simulink model "hexapod"  (R2015a)
settings: Solver=ode23tb  StartTime=0.0  StopTime=10  FixedStep=0.001  MaxStep=0.01  RelTol=1e-4  AbsTol=1e-5
values from neighbouring files (symbols this model uses):
  bL = 18.5    [runFirst.m]    (also in runFirst2.m = 20.5)
  bWb = 12.5    [runFirst.m]    (also in runFirst2.m = 14.5)
  bWs = 10.5    [runFirst.m]    (also in runFirst2.m = 12.5)
  C = CM + CL/n^2    (= 0.0001377500155)    [runFirst.m]
  d1 = 0    [runFirst.m]    (also in runFirst2.m)
  d2 = -4.61    [runFirst.m]    (also in runFirst2.m = 0)
  J = JM + JL/n^2    (= 0.008455500031)    [runFirst.m]
  Ka = 12    [runFirst.m]
  Kb = 0.00867    [runFirst.m]
  Ke = 1    [runFirst.m]
  Km = 4.375    [runFirst.m]
  L = 0.0006    [runFirst.m]
  L1 = 3.64    [runFirst.m]    (also in runFirst2.m = 3.4)
  l1x = 15.78    [runFirst.m]
  l1y = 11.78    [runFirst.m]
  l1z = -14.9    [runFirst.m]
  L2 = 5.72    [runFirst.m]    (also in runFirst2.m = 8.7)
  l2x = 0    [runFirst.m]
  l2y = 15.48    [runFirst.m]
  l2z = -14.9    [runFirst.m]
  L3 = 12.46    [runFirst.m]    (also in runFirst2.m = 12.73)
  l3x = -15.78    [runFirst.m]
  l3y = 11.78    [runFirst.m]
  l3z = -14.9    [runFirst.m]
  l4x = 15.78    [runFirst.m]
  l4y = -11.78    [runFirst.m]
  l4z = -14.9    [runFirst.m]
  l5x = 0    [runFirst.m]
  l5y = -15.48    [runFirst.m]
  l5z = -14.9    [runFirst.m]
  l6x = -15.78    [runFirst.m]
  l6y = -11.78    [runFirst.m]
  l6z = -14.9    [runFirst.m]
  n = 254    [runFirst.m]
  R = 1.4    [runFirst.m]
  stX = 4    [runFirst.m]
  stZ = 2    [runFirst.m]
  Ts = 2    [runFirst.m]
undefined symbols (not defined in the file or in its folder): X, Y, Z
undefined symbols (not defined in the file): bH, bM, m1, m2, m3
libraries: sm_lib x108, nesl_utility x52, simulink x12, Contact_Forces_Lib x7, roblocks x2
(part 1 of 5)
settings Model: Creator=340DANILOV  LastModifiedBy=340DANILOV
settings SolverCC: ZeroCrossAlgorithm=Adaptive
settings DataIOCC: LimitDataPoints=off  ReturnWorkspaceOutputs=on
settings DebuggingCC: IgnoredZcDiagnostic=none  SolverPrmCheckMsg=warning  UnconnectedInputMsg=none  UnconnectedOutputMsg=none
settings DiagnosticsConfigSet: SimMechanicsRigidlyBoundBlock=none

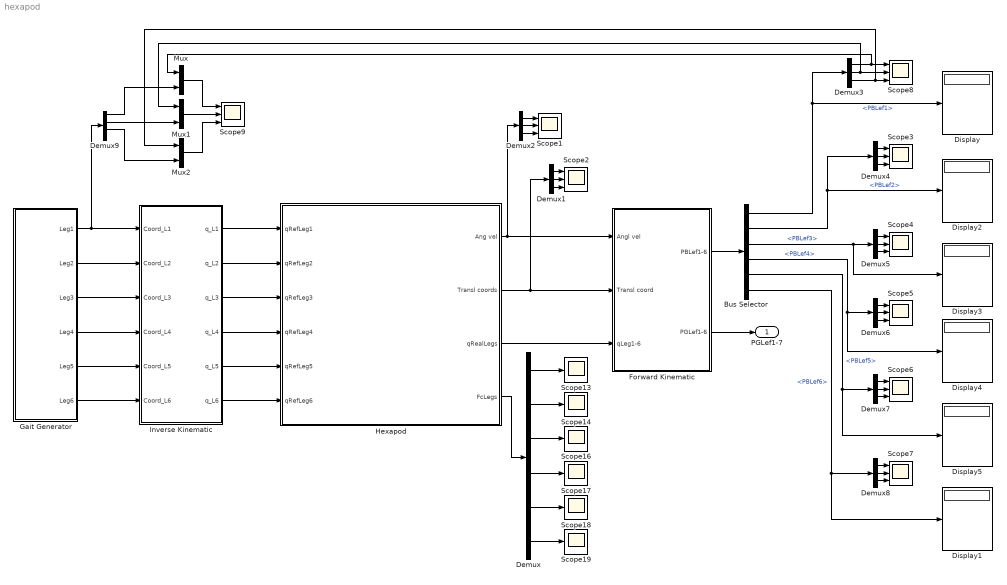
== system hexapod ==
  Bus Selector : BusSelector  OutputSignals=PBLef1,PBLef2,PBLef3,PBLef4,PBLef5,PBLef6
  Demux : Demux  Outputs=6
  Demux{1..8} (8 alike) : Demux  Outputs=3
  Demux9 : Demux
  Display{,1..5} (6 alike) : Display
  Forward Kinematic : Subsystem
  Gait Generator : Subsystem
  Hexapod : Subsystem  mask(Hexapod model){bLength=bL, bSmWidth=bWs, bBigWidth=bWb, bHeight=bH, bMass=bM, L1Length=L1, L2Length=L2, L3Length=L3, L1Mass=m1, L2Mass=m2, L3Mass=m3, dirAngle=45, GsurfX=10, GsurfY=1}
      mask prompts: bLength "Length [cm]"; bSmWidth "Small Width  [cm]"; bBigWidth "Big Width  [cm]"; bHeight "Height  [cm]"; bMass "Mass [kg]"; L1Length "Link 1"; L2Length "Link 2"; L3Length "Link3"; L1Mass "Link 1"; L2Mass "Link 2"; L3Mass "Link 3"; dirAngle "Angle of legs direction relative to body [grad]"; GsurfX "X"; GsurfY "Y"
      mask help:
      | This model describes hexapod robot with six insect legs. This model contain mechanics and servos.
      | You can change mass and size charasteristics of body and legs.
      | As a location is used a flat surface.
      |
      | Inputs:
      |  - qRefLeg<1...6> - reference angles for each leg.
      |             It is must be 1x3 massive with angles for each joint of leg.
      |
      | Outputs:
      |  - Ang vel - Angular velocities of CoM. Imitation of data from gyroscope.
      |  - Transl accel - CoM translation acceleration. Imitation of data from accelerometer.
      |  - FcLegs - Contact forces of end effectors each leg. It is 1x6 massive. Each element contains value for contact force each leg. Imitation of force sensors.
      |  - qRealLegs - Real angles of each link of hexapod legs. It is 3x6 massive. Imitation of data from servo encoder.
      mask DialogControl Control2 Prompt: You can customize parameters of the hexapod body here.
      mask DialogControl Container8 Prompt: Length of links [cm]
      mask DialogControl Container14 Prompt: Mass of links [kg]
      mask DialogControl Control6 Prompt: Enter parameters of surface geometry [m].
      mask Display:
      | image(imread('hexapod.png'))
      | 
      | 
      | port_label('output',1,'Ang vel')
      | port_label('output',2,'Transl accel')
      | port_label('output',3,'qRealLegs')
      | port_label('output',4,'FcLegs')
      | 
      | port_label('input',1,'qRefLeg1')
      | port_label('input',2,'qRefLeg2')
      | port_label('input',3,'qRefLeg3')
      | port_label('input',4,'qRefLeg4')
      | port_label('input',5,'qRefLeg5')
      | port_label('input',6,'qRefLeg6')
  Inverse Kinematic : Subsystem
  Mux : Mux  Inputs=2
  Mux1 : Mux  Inputs=2
  Mux2 : Mux  Inputs=2
  Scope{1..9} (9 alike) : Scope  NumInputPorts=3
      Scope1 settings: YMin=-15~-5~-5  YMax=20~5~5  SaveName=ScopeData22
      Scope2 settings: YMin=-15~-5~-5  YMax=20~5~5  SaveName=ScopeData25
      Scope3 settings: YMin=-15~-5~-5  YMax=20~5~5  SaveName=ScopeData32
      Scope4 settings: YMin=-15~-5~-5  YMax=20~5~5  SaveName=ScopeData33
      Scope5 settings: YMin=-15~-5~-5  YMax=20~5~5  SaveName=ScopeData34
      Scope6 settings: YMin=-15~-5~-5  YMax=20~5~5  SaveName=ScopeData35
      Scope7 settings: YMin=-15~-5~-5  YMax=20~5~5  SaveName=ScopeData36
      Scope8 settings: YMin=-15~-5~-5  YMax=20~5~5  SaveName=ScopeData44
      Scope9 settings: YMin=-15~10.5~-5  YMax=20~13~5  SaveName=ScopeData37
  Scope{13..14,16..19} (6 alike) : Scope
      Scope13 settings: SaveName=ScopeData23
      Scope14 settings: SaveName=ScopeData24
      Scope16 settings: SaveName=ScopeData26
      Scope17 settings: SaveName=ScopeData27
      Scope18 settings: SaveName=ScopeData28
      Scope19 settings: SaveName=ScopeData29
  PGLef1-7 : Outport
  wires:
  Hexapod/4(FcLegs) -> Demux/1
  Hexapod/1(Ang vel) -> Demux2/1, Forward Kinematic/1(Angl vel)
  Hexapod/2(Transl coords) -> Demux1/1, Forward Kinematic/2(Transl coord)
  Hexapod/3(qRealLegs) -> Forward Kinematic/3(qLeg1-6)
  Forward Kinematic/1(PBLef1-6) -> Bus Selector/1
  Forward Kinematic/2(PGLef1-6) -> PGLef1-7/1
  Bus Selector/1 -> Demux3/1, Display/1  "<PBLef1>"
  Bus Selector/6 -> Demux8/1, Display1/1  "<PBLef6>"
  Bus Selector/2 -> Demux4/1, Display2/1  "<PBLef2>"
  Bus Selector/3 -> Demux5/1, Display3/1  "<PBLef3>"
  Bus Selector/4 -> Demux6/1, Display4/1  "<PBLef4>"
  Bus Selector/5 -> Demux7/1, Display5/1  "<PBLef5>"
  Gait Generator/2(Leg2) -> Inverse Kinematic/2(Coord_L2)
  Gait Generator/1(Leg1) -> Demux9/1, Inverse Kinematic/1(Coord_L1)
  Gait Generator/3(Leg3) -> Inverse Kinematic/3(Coord_L3)
  Gait Generator/4(Leg4) -> Inverse Kinematic/4(Coord_L4)
  Gait Generator/5(Leg5) -> Inverse Kinematic/5(Coord_L5)
  Gait Generator/6(Leg6) -> Inverse Kinematic/6(Coord_L6)
  Inverse Kinematic/2(q_L2) -> Hexapod/2(qRefLeg2)
  Inverse Kinematic/1(q_L1) -> Hexapod/1(qRefLeg1)
  Inverse Kinematic/3(q_L3) -> Hexapod/3(qRefLeg3)
  Inverse Kinematic/4(q_L4) -> Hexapod/4(qRefLeg4)
  Inverse Kinematic/5(q_L5) -> Hexapod/5(qRefLeg5)
  Inverse Kinematic/6(q_L6) -> Hexapod/6(qRefLeg6)
  Demux/1 -> Scope13/1
  Demux/2 -> Scope14/1
  Demux/3 -> Scope16/1
  Demux/4 -> Scope17/1
  Demux/5 -> Scope18/1
  Demux/6 -> Scope19/1
  Demux2/3 -> Scope1/3
  Demux2/2 -> Scope1/2
  Demux2/1 -> Scope1/1
  Demux1/3 -> Scope2/3
  Demux1/2 -> Scope2/2
  Demux1/1 -> Scope2/1
  Demux3/1 -> Scope8/1, Mux/1
  Demux4/3 -> Scope3/3
  Demux4/2 -> Scope3/2
  Demux4/1 -> Scope3/1
  Demux5/3 -> Scope4/3
  Demux5/2 -> Scope4/2
  Demux5/1 -> Scope4/1
  Demux6/3 -> Scope5/3
  Demux6/2 -> Scope5/2
  Demux6/1 -> Scope5/1
  Demux7/3 -> Scope6/3
  Demux7/2 -> Scope6/2
  Demux7/1 -> Scope6/1
  Demux8/3 -> Scope7/3
  Demux8/2 -> Scope7/2
  Demux8/1 -> Scope7/1
  Demux9/1 -> Mux/2
  Demux9/2 -> Mux1/2
  Demux9/3 -> Mux2/2
  Demux3/2 -> Scope8/2, Mux1/1
  Demux3/3 -> Scope8/3, Mux2/1
  Mux1/1 -> Scope9/2
  Mux/1 -> Scope9/1
  Mux2/1 -> Scope9/3

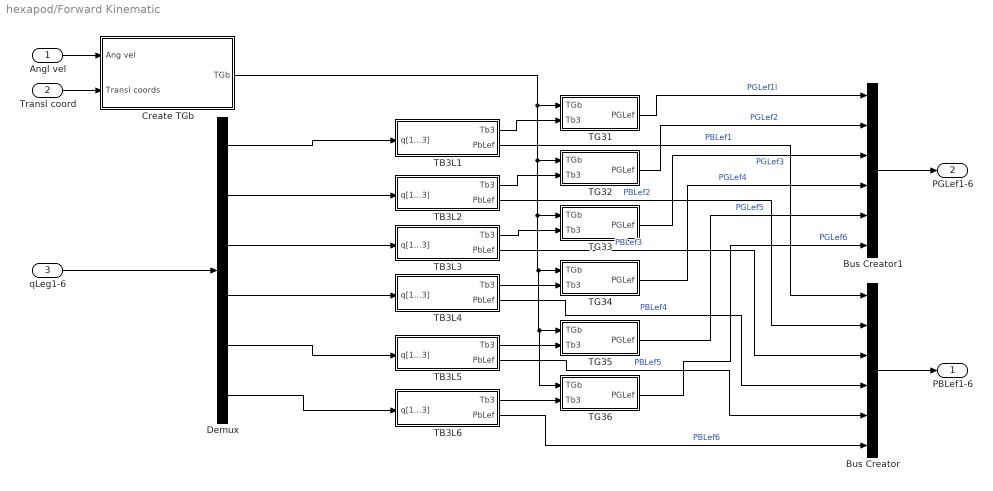
== system hexapod/Forward Kinematic ==
  Angl vel : Inport
  Transl coord : Inport  Port=2
  qLeg1-6 : Inport  Port=3
  Bus Creator : BusCreator  Inputs=6
  Bus Creator1 : BusCreator  Inputs=6
  Create TGb : Subsystem
  Demux : Demux  Outputs=6
  TB3L1 : Subsystem
  TB3L2 : Subsystem
  TB3L3 : Subsystem
  TB3L4 : Subsystem
  TB3L5 : Subsystem
  TB3L6 : Subsystem
  TG31 : Subsystem
  TG32 : Subsystem
  TG33 : Subsystem
  TG34 : Subsystem
  TG35 : Subsystem
  TG36 : Subsystem
  PBLef1-6 : Outport
  PGLef1-6 : Outport  Port=2
  wires:
  Bus Creator/1 -> PBLef1-6/1
  TB3L6/1(Tb3) -> TG36/2(Tb3)
  TB3L5/2(PbLef) -> Bus Creator/5  "PBLef5"
  TB3L4/2(PbLef) -> Bus Creator/4  "PBLef4"
  TG35/1(PGLef) -> Bus Creator1/5  "PGLef5"
  TB3L6/2(PbLef) -> Bus Creator/6  "PBLef6"
  Demux/1 -> TB3L1/1(q[1...3])
  TB3L1/2(PbLef) -> Bus Creator/1  "PBLef1"
  Demux/6 -> TB3L6/1(q[1...3])
  TB3L1/1(Tb3) -> TG31/2(Tb3)
  Create TGb/1(TGb) -> TG36/1(TGb), TG35/1(TGb), TG34/1(TGb), TG33/1(TGb), TG32/1(TGb), TG31/1(TGb)
  Demux/4 -> TB3L4/1(q[1...3])
  Demux/3 -> TB3L3/1(q[1...3])
  TG31/1(PGLef) -> Bus Creator1/1  "PGLef1l"
  Demux/5 -> TB3L5/1(q[1...3])
  TB3L2/2(PbLef) -> Bus Creator/2  "PBLef2"
  TB3L2/1(Tb3) -> TG32/2(Tb3)
  TG32/1(PGLef) -> Bus Creator1/2  "PGLef2"
  TB3L4/1(Tb3) -> TG34/2(Tb3)
  TB3L3/1(Tb3) -> TG33/2(Tb3)
  TG33/1(PGLef) -> Bus Creator1/3  "PGLef3"
  Bus Creator1/1 -> PGLef1-6/1
  Angl vel/1 -> Create TGb/1(Ang vel)
  Transl coord/1 -> Create TGb/2(Transl coords)
  TB3L3/2(PbLef) -> Bus Creator/3  "PBLef3"
  qLeg1-6/1 -> Demux/1
  TB3L5/1(Tb3) -> TG35/2(Tb3)
  TG36/1(PGLef) -> Bus Creator1/6  "PGLef6"
  TG34/1(PGLef) -> Bus Creator1/4  "PGLef4"
  Demux/2 -> TB3L2/1(q[1...3])

== system hexapod/Gait Generator ==
  Leg1_xyz : Subsystem
  Leg2_xyz : Subsystem
  Leg3_xyz : Subsystem
  Leg4_xyz : Subsystem
  Leg5_xyz : Subsystem
  Leg6_xyz : Subsystem
  Leg1 : Outport
  Leg2 : Outport  Port=2
  Leg3 : Outport  Port=3
  Leg4 : Outport  Port=4
  Leg5 : Outport  Port=5
  Leg6 : Outport  Port=6
  wires:
  Leg6_xyz/1(Out1) -> Leg6/1
  Leg1_xyz/1(Out1) -> Leg1/1
  Leg5_xyz/1(Out1) -> Leg5/1
  Leg3_xyz/1(Out1) -> Leg3/1
  Leg2_xyz/1(Out1) -> Leg2/1
  Leg4_xyz/1(Out1) -> Leg4/1

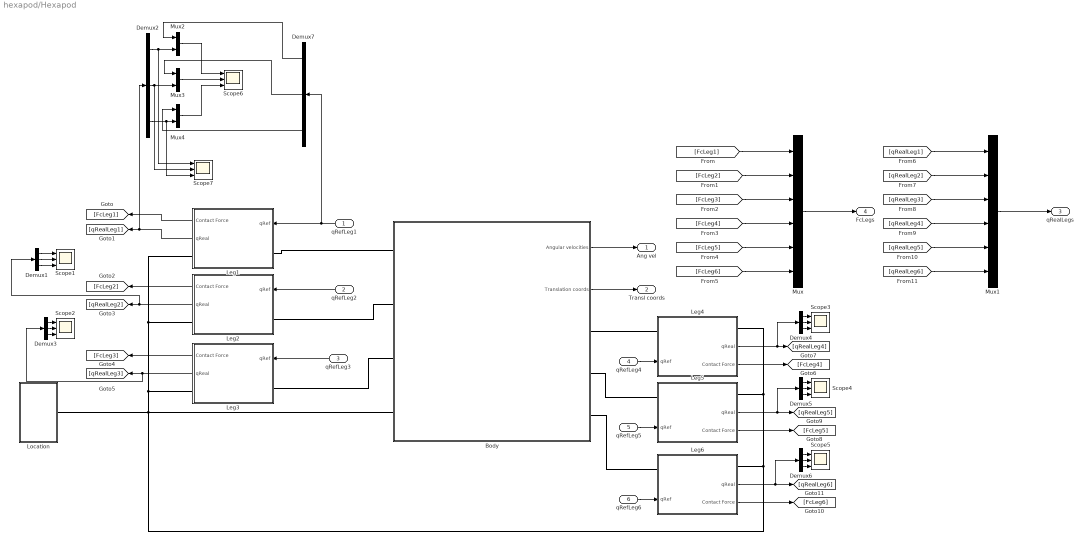
== system hexapod/Hexapod ==
  qRefLeg1 : Inport
  qRefLeg2 : Inport  Port=2
  qRefLeg3 : Inport  Port=3
  qRefLeg4 : Inport  Port=4
  qRefLeg5 : Inport  Port=5
  qRefLeg6 : Inport  Port=6
  Body : Subsystem  mask(Hexapod Body){L=bLength, w1=bSmWidth, w2=bBigWidth, H=bHeight, m=bMass, Z1Angle=dirAngle, Z2Angle=0, Z3Angle=-dirAngle, Z4Angle=-dirAngle, Z5Angle=0, Z6Angle=dirAngle}
      mask prompts: L "Length (cm)"; w1 "Small weigth (cm)"; w2 "Big weigth (cm)"; H "Heigth (cm)"; m "Mass (kg)"; Z1Angle "Leg1 Rotation"; Z2Angle "Leg2 Rotation"; Z3Angle "Leg3 Rotation"; Z4Angle "Leg4 Rotation"; Z5Angle "Leg5 Rotation"; Z6Angle "Leg6 Rotation"
      mask help: This block describes overall size, mass and reference frames of hexapod body.
      mask Display:
      | image(imread('body.png'))
      | text(5,10, 'Hexapod Body')
      | port_label('LConn',1,'Leg1')
      | port_label('LConn',2,'Leg2')
      | port_label('LConn',3,'Leg3')
      | port_label('LConn',4,'Global System')
      | port_label('RConn',1,'Leg4')
      | port_label('RConn',2,'Leg5')
      | port_label('RConn',3,'Leg6')
      | port_label('output',1,'Ang vel')
      | port_label('output',2,'Transl accel')
  Demux{1..7} (7 alike) : Demux  Outputs=3
  Leg1 : Subsystem  mask(Insect leg){L1=L1Length, L2=L2Length, L3=L3Length, m1=L1Mass, m2=L2Mass, m3=L3Mass}
      mask prompts: L1 "Length 1 (cm)"; L2 "Lengh 2 (cm)"; L3 "Length 3 (cm)"; m1 "Mass 1 (kg)"; m2 "Mass 2 (kg)"; m3 "Mass 3(kg)"
      mask help: This block describes link length and their mass of the hexapod insect leg.
      mask Display:
      | image(imread('insect_leg.png'))
      | text(5,10, 'Insect leg')
      | port_label('LConn',1,'T0')
      | port_label('RConn',1,'Base')
      | port_label('input',1,'qRef')
      | port_label('output',1,'Fc')
      | port_label('output',2,'qReal')
  Leg2 : Subsystem  mask(Insect leg){L1=L1Length, L2=L2Length, L3=L3Length, m1=L1Mass, m2=L2Mass, m3=L3Mass}
      mask prompts: L1 "Length 1 (cm)"; L2 "Lengh 2 (cm)"; L3 "Length 3 (cm)"; m1 "Mass 1 (kg)"; m2 "Mass 2 (kg)"; m3 "Mass 3(kg)"
      mask help: This block describes link length and their mass of the hexapod insect leg.
      mask Display:
      | image(imread('insect_leg.png'))
      | text(5,10, 'Insect leg')
      | port_label('LConn',1,'T0')
      | port_label('RConn',1,'Base')
      | port_label('input',1,'qRef')
      | port_label('output',1,'Fc')
      | port_label('output',2,'qReal')
  Leg3 : Subsystem  mask(Insect leg){L1=L1Length, L2=L2Length, L3=L3Length, m1=L1Mass, m2=L2Mass, m3=L3Mass}
      mask prompts: L1 "Length 1 (cm)"; L2 "Lengh 2 (cm)"; L3 "Length 3 (cm)"; m1 "Mass 1 (kg)"; m2 "Mass 2 (kg)"; m3 "Mass 3(kg)"
      mask help: This block describes link length and their mass of the hexapod insect leg.
      mask Display:
      | image(imread('insect_leg.png'))
      | text(5,10, 'Insect leg')
      | port_label('LConn',1,'T0')
      | port_label('RConn',1,'Base')
      | port_label('input',1,'qRef')
      | port_label('output',1,'Fc')
      | port_label('output',2,'qReal')
  Leg4 : Subsystem  mask(Insect leg){L1=L1Length, L2=L2Length, L3=L3Length, m1=L1Mass, m2=L2Mass, m3=L3Mass}
      mask prompts: L1 "Length 1 (cm)"; L2 "Lengh 2 (cm)"; L3 "Length 3 (cm)"; m1 "Mass 1 (kg)"; m2 "Mass 2 (kg)"; m3 "Mass 3(kg)"
      mask help: This block describes link length and their mass of the hexapod insect leg.
      mask Display:
      | image(imread('insect_leg.png'))
      | text(5,10, 'Insect leg')
      | port_label('LConn',1,'T0')
      | port_label('RConn',1,'Base')
      | port_label('input',1,'qRef')
      | port_label('output',1,'Fc')
      | port_label('output',2,'qReal')
  Leg5 : Subsystem  mask(Insect leg){L1=L1Length, L2=L2Length, L3=L3Length, m1=L1Mass, m2=L2Mass, m3=L3Mass}
      mask prompts: L1 "Length 1 (cm)"; L2 "Lengh 2 (cm)"; L3 "Length 3 (cm)"; m1 "Mass 1 (kg)"; m2 "Mass 2 (kg)"; m3 "Mass 3(kg)"
      mask help: This block describes link length and their mass of the hexapod insect leg.
      mask Display:
      | image(imread('insect_leg.png'))
      | text(5,10, 'Insect leg')
      | port_label('LConn',1,'T0')
      | port_label('RConn',1,'Base')
      | port_label('input',1,'qRef')
      | port_label('output',1,'Fc')
      | port_label('output',2,'qReal')
  Leg6 : Subsystem  mask(Insect leg){L1=L1, L2=L2, L3=L3, m1=m1, m2=m2, m3=m3}
      mask prompts: L1 "Length 1 (cm)"; L2 "Lengh 2 (cm)"; L3 "Length 3 (cm)"; m1 "Mass 1 (kg)"; m2 "Mass 2 (kg)"; m3 "Mass 3(kg)"
      mask help: This block describes link length and their mass of the hexapod insect leg.
      mask Display:
      | image(imread('insect_leg.png'))
      | text(5,10, 'Insect leg')
      | port_label('LConn',1,'T0')
      | port_label('RConn',1,'Base')
      | port_label('input',1,'qRef')
      | port_label('output',1,'Fc')
      | port_label('output',2,'qReal')
  Location : Subsystem
  Mux : Mux  Inputs=6
  Mux1 : Mux  Inputs=6
  Mux2 : Mux  Inputs=2
  Mux3 : Mux  Inputs=2
  Mux4 : Mux  Inputs=2
  Scope{1..7} (7 alike) : Scope  NumInputPorts=3
      Scope1 settings: YMin=-15~-5~-5  YMax=20~5~5  SaveName=ScopeData17
      Scope2 settings: YMin=-15~-5~-5  YMax=20~5~5  SaveName=ScopeData18
      Scope3 settings: YMin=-15~-5~-5  YMax=20~5~5  SaveName=ScopeData19
      Scope4 settings: YMin=-15~-5~-5  YMax=20~5~5  SaveName=ScopeData20
      Scope5 settings: YMin=-15~-5~-5  YMax=20~5~5  SaveName=ScopeData21
      Scope6 settings: YMin=-15~-5~-5  YMax=20~5~5  SaveName=ScopeData16
      Scope7 settings: YMin=-15~-5~-5  YMax=20~5~5  SaveName=ScopeData50
  Ang vel : Outport
  Transl coords : Outport  Port=2
  qRealLegs : Outport  Port=3
  FcLegs : Outport  Port=4
  wires:
  qRefLeg1/1 -> Demux7/1, Leg1/1(qRef)
  qRefLeg2/1 -> Leg2/1(qRef)
  qRefLeg3/1 -> Leg3/1(qRef)
  qRefLeg4/1 -> Leg4/1(qRef)
  Leg2/2(qReal) -> Demux1/1, [qRealLeg2]
  Leg3/2(qReal) -> Demux3/1, [qRealLeg3]
  Leg3/1(Contact Force) -> [FcLeg3]
  [FcLeg2] -> Mux/2
  [FcLeg4] -> Mux/4
  [FcLeg5] -> Mux/5
  [FcLeg1] -> Mux/1
  [FcLeg3] -> Mux/3
  [FcLeg6] -> Mux/6
  Mux/1 -> FcLegs/1
  Leg1/1(Contact Force) -> [FcLeg1]
  [qRealLeg4] -> Mux1/4
  [qRealLeg6] -> Mux1/6
  [qRealLeg2] -> Mux1/2
  [qRealLeg1] -> Mux1/1
  Mux1/1 -> qRealLegs/1
  [qRealLeg5] -> Mux1/5
  [qRealLeg3] -> Mux1/3
  Body/1(Angular velocities) -> Ang vel/1
  Body/2(Translation coords) -> Transl coords/1
  Leg1/2(qReal) -> Demux2/1, [qRealLeg1]
  Leg2/1(Contact Force) -> [FcLeg2]
  qRefLeg5/1 -> Leg5/1(qRef)
  qRefLeg6/1 -> Leg6/1(qRef)
  Leg4/1(Contact Force) -> [FcLeg4]
  Leg4/2(qReal) -> Demux4/1, [qRealLeg4]
  Leg5/2(qReal) -> Demux5/1, [qRealLeg5]
  Leg5/1(Contact Force) -> [FcLeg5]
  Leg6/2(qReal) -> Demux6/1, [qRealLeg6]
  Leg6/1(Contact Force) -> [FcLeg6]
  Demux1/3 -> Scope1/3
  Demux1/2 -> Scope1/2
  Demux1/1 -> Scope1/1
  Demux3/3 -> Scope2/3
  Demux3/2 -> Scope2/2
  Demux3/1 -> Scope2/1
  Demux4/3 -> Scope3/3
  Demux4/2 -> Scope3/2
  Demux4/1 -> Scope3/1
  Demux5/3 -> Scope4/3
  Demux5/2 -> Scope4/2
  Demux5/1 -> Scope4/1
  Demux6/3 -> Scope5/3
  Demux6/2 -> Scope5/2
  Demux6/1 -> Scope5/1
  Demux2/1 -> Scope7/1, Mux2/2
  Demux2/2 -> Scope7/2, Mux3/2
  Demux2/3 -> Scope7/3, Mux4/2
  Mux3/1 -> Scope6/2
  Mux2/1 -> Scope6/1
  Mux4/1 -> Scope6/3
  Demux7/1 -> Mux2/1
  Demux7/2 -> Mux3/1
  Demux7/3 -> Mux4/1
  connections:
  Body/LConn1 -- Leg1/LConn1
  Body/LConn4 -- Leg6/RConn1 -- Leg5/RConn1 -- Leg4/RConn1 -- Location/RConn1 -- Leg3/RConn1 -- Leg2/RConn1 -- Leg1/RConn1
  Leg2/LConn1 -- Body/LConn2
  Leg3/LConn1 -- Body/LConn3
  Leg4/LConn1 -- Body/RConn1
  Leg5/LConn1 -- Body/RConn2
  Leg6/LConn1 -- Body/RConn3

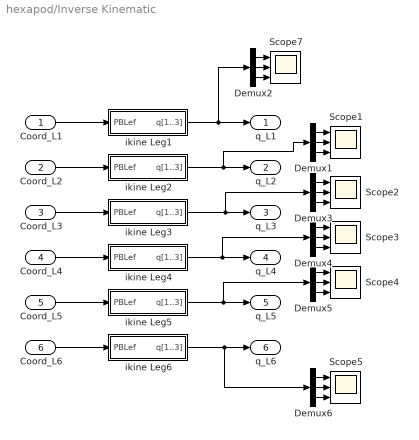
== system hexapod/Inverse Kinematic ==
  Coord_L1 : Inport
  Coord_L2 : Inport  Port=2
  Coord_L3 : Inport  Port=3
  Coord_L4 : Inport  Port=4
  Coord_L5 : Inport  Port=5
  Coord_L6 : Inport  Port=6
  Demux{1..6} (6 alike) : Demux  Outputs=3
  Scope{1..5,7} (6 alike) : Scope  NumInputPorts=3
      Scope1 settings: YMin=-15~-5~-5  YMax=20~5~5  SaveName=ScopeData9
      Scope2 settings: YMin=-15~-5~-5  YMax=20~5~5  SaveName=ScopeData11
      Scope3 settings: YMin=-15~-5~-5  YMax=20~5~5  SaveName=ScopeData12
      Scope4 settings: YMin=-15~-5~-5  YMax=20~5~5  SaveName=ScopeData13
      Scope5 settings: YMin=-15~-5~-5  YMax=20~5~5  SaveName=ScopeData14
      Scope7 settings: YMin=-15~-5~-5  YMax=20~5~5  SaveName=ScopeData39
  ikine Leg1 : Subsystem
  ikine Leg2 : Subsystem
  ikine Leg3 : Subsystem
  ikine Leg4 : Subsystem
  ikine Leg5 : Subsystem
  ikine Leg6 : Subsystem
  q_L1 : Outport
  q_L2 : Outport  Port=2
  q_L3 : Outport  Port=3
  q_L4 : Outport  Port=4
  q_L5 : Outport  Port=5
  q_L6 : Outport  Port=6
  wires:
  ikine Leg1/1(q[1..3]) -> Demux2/1, q_L1/1
  ikine Leg2/1(q[1..3]) -> Demux1/1, q_L2/1
  ikine Leg3/1(q[1..3]) -> Demux3/1, q_L3/1
  ikine Leg4/1(q[1..3]) -> Demux4/1, q_L4/1
  ikine Leg5/1(q[1..3]) -> Demux5/1, q_L5/1
  ikine Leg6/1(q[1..3]) -> Demux6/1, q_L6/1
  Coord_L1/1 -> ikine Leg1/1(PBLef)
  Coord_L2/1 -> ikine Leg2/1(PBLef)
  Coord_L3/1 -> ikine Leg3/1(PBLef)
  Coord_L4/1 -> ikine Leg4/1(PBLef)
  Coord_L5/1 -> ikine Leg5/1(PBLef)
  Coord_L6/1 -> ikine Leg6/1(PBLef)
  Demux2/3 -> Scope7/3
  Demux2/2 -> Scope7/2
  Demux2/1 -> Scope7/1
  Demux1/3 -> Scope1/3
  Demux1/2 -> Scope1/2
  Demux1/1 -> Scope1/1
  Demux3/3 -> Scope2/3
  Demux3/2 -> Scope2/2
  Demux3/1 -> Scope2/1
  Demux4/3 -> Scope3/3
  Demux4/2 -> Scope3/2
  Demux4/1 -> Scope3/1
  Demux5/3 -> Scope4/3
  Demux5/2 -> Scope4/2
  Demux5/1 -> Scope4/1
  Demux6/3 -> Scope5/3
  Demux6/2 -> Scope5/2
  Demux6/1 -> Scope5/1

== system hexapod/Forward Kinematic/Create TGb ==
  note: TBG
  Ang vel : Inport
  Transl coords : Inport  Port=2
  Demux : Demux  Outputs=3
  Demux1 : Demux  Outputs=3
  Gain : Gain  Gain=-1
  Gain1 : Gain  Gain=-1
  Gain2 : Gain  Gain=-1
  Integrator : Integrator
  Integrator1 : Integrator
  Integrator2 : Integrator
  Product : Product  Multiplication=Matrix(*)
  Scope1 : Scope  NumInputPorts=3
      settings: YMin=-15~-5~-5  YMax=20~5~5  SaveName=ScopeData38
  Scope6 : Scope  NumInputPorts=3
      settings: YMin=-15~-5~-5  YMax=20~5~5  SaveName=ScopeData48
  Switch1 : Subsystem
  Switch2 : Subsystem
  rpy2T : roblocks/Transform Conversion/rpy2T
      link override MATLAB Fcn: MATLABFcn=rpy2tr(u(1),u(2),u(3))
  xyz2T : roblocks/Transform Conversion/xyz2T
  TGb : Outport
  wires:
  Integrator1/1 -> Scope6/2, rpy2T/2
  Integrator2/1 -> Scope6/3, rpy2T/3
  Integrator/1 -> Scope6/1, rpy2T/1
  Switch2/1(Out1) -> Demux1/1
  Transl coords/1 -> Switch2/1(In1)
  Ang vel/1 -> Switch1/1(In1)
  Switch1/1(Out1) -> Demux/1
  Demux1/1 -> Gain/1
  Demux1/2 -> Gain1/1
  Demux1/3 -> Gain2/1
  Demux/3 -> Integrator2/1
  Product/1 -> TGb/1
  xyz2T/1 -> Product/2
  rpy2T/1 -> Product/1
  Demux/2 -> Integrator1/1
  Demux/1 -> Integrator/1
  Gain/1 -> Scope1/1, xyz2T/1
  Gain1/1 -> xyz2T/2, Scope1/2
  Gain2/1 -> xyz2T/3, Scope1/3

== system hexapod/Forward Kinematic/TB3L1 ==
  note: Tb3
  note: PBL1ef
  q[1...3] : Inport
  Constant : Constant  Value=[L3; 0; 0; 1]  VectorParams1D=off
  Demux2 : Demux
  Mux : Mux  Inputs=3
  Product1 : Product  Multiplication=Matrix(*)
  Product2 : Product  Multiplication=Matrix(*)
  T30 : Subsystem
  Tbleg1 : Constant  Value=[cos(45*pi/180) -sin(45*pi/180) 0 bL/2; sin(45*pi/180) cos(45*pi/180) 0 bWs/2; 0 0 1 0; 0 0 0 1]  VectorParams1D=off
  Terminator : Terminator
  Tb3 : Outport
  PbLef : Outport  Port=2
  wires:
  Constant/1 -> Product1/2
  q[1...3]/1 -> T30/1(In1)
  T30/1(Out1) -> Product2/2
  Tbleg1/1 -> Product2/1
  Demux2/3 -> Mux/3
  Product1/1 -> Demux2/1
  Demux2/4 -> Terminator/1
  Demux2/1 -> Mux/1
  Mux/1 -> PbLef/1
  Demux2/2 -> Mux/2
  Product2/1 -> Tb3/1, Product1/1

== system hexapod/Forward Kinematic/TB3L2 ==
  note: PBL1ef
  note: Tb3
  q[1...3] : Inport
  Constant : Constant  Value=[L3; 0; 0; 1]  VectorParams1D=off
  Demux2 : Demux
  Mux : Mux  Inputs=3
  Product1 : Product  Multiplication=Matrix(*)
  Product2 : Product  Multiplication=Matrix(*)
  T30 : Subsystem
  Tbleg1 : Constant  Value=[0 -1 0 0; 1 0 0 bWb/2; 0 0 1 0; 0 0 0 1]  VectorParams1D=off
  Terminator : Terminator
  Tb3 : Outport
  PbLef : Outport  Port=2
  wires:
  Product2/1 -> Product1/1, Tb3/1
  Demux2/2 -> Mux/2
  Mux/1 -> PbLef/1
  Demux2/1 -> Mux/1
  Demux2/4 -> Terminator/1
  Product1/1 -> Demux2/1
  Demux2/3 -> Mux/3
  Tbleg1/1 -> Product2/1
  T30/1(Out1) -> Product2/2
  q[1...3]/1 -> T30/1(In1)
  Constant/1 -> Product1/2

== system hexapod/Forward Kinematic/TB3L3 ==
  note: Tb3
  note: PBL1ef
  q[1...3] : Inport
  Constant : Constant  Value=[L3; 0; 0; 1]  VectorParams1D=off
  Demux2 : Demux
  Mux : Mux  Inputs=3
  Product1 : Product  Multiplication=Matrix(*)
  Product2 : Product  Multiplication=Matrix(*)
  T30 : Subsystem
  Tbleg3 : Constant  Value=[cos(135*pi/180) -sin(135*pi/180) 0 -bL/2; sin(135*pi/180) cos(135*pi/180) 0 bWs/2; 0 0 1 0; 0 0 0 1]  VectorParams1D=off
  Terminator : Terminator
  Tb3 : Outport
  PbLef : Outport  Port=2
  wires:
  Constant/1 -> Product1/2
  q[1...3]/1 -> T30/1(In1)
  T30/1(Out1) -> Product2/2
  Tbleg3/1 -> Product2/1
  Demux2/3 -> Mux/3
  Product1/1 -> Demux2/1
  Demux2/4 -> Terminator/1
  Demux2/1 -> Mux/1
  Mux/1 -> PbLef/1
  Demux2/2 -> Mux/2
  Product2/1 -> Tb3/1, Product1/1

== system hexapod/Forward Kinematic/TB3L4 ==
  note: PBL1ef
  note: Tb3
  q[1...3] : Inport
  Constant : Constant  Value=[L3; 0; 0; 1]  VectorParams1D=off
  Demux2 : Demux
  Mux : Mux  Inputs=3
  Product1 : Product  Multiplication=Matrix(*)
  Product2 : Product  Multiplication=Matrix(*)
  T30 : Subsystem
  Tbleg1 : Constant  Value=[cos(-45*pi/180) -sin(-45*pi/180) 0 bL/2; sin(-45*pi/180) cos(-45*pi/180) 0 -bWs/2; 0 0 1 0; 0 0 0 1]  VectorParams1D=off
  Terminator : Terminator
  Tb3 : Outport
  PbLef : Outport  Port=2
  wires:
  Product2/1 -> Product1/1, Tb3/1
  Demux2/2 -> Mux/2
  Mux/1 -> PbLef/1
  Demux2/1 -> Mux/1
  Demux2/4 -> Terminator/1
  Product1/1 -> Demux2/1
  Demux2/3 -> Mux/3
  Tbleg1/1 -> Product2/1
  T30/1(Out1) -> Product2/2
  q[1...3]/1 -> T30/1(In1)
  Constant/1 -> Product1/2

== system hexapod/Forward Kinematic/TB3L5 ==
  note: Tb3
  note: PBL1ef
  q[1...3] : Inport
  Constant : Constant  Value=[L3; 0; 0; 1]  VectorParams1D=off
  Demux2 : Demux
  Mux : Mux  Inputs=3
  Product1 : Product  Multiplication=Matrix(*)
  Product2 : Product  Multiplication=Matrix(*)
  T30 : Subsystem
  Tbleg1 : Constant  Value=[0 1 0 0; -1 0 0 -bWb/2; 0 0 1 0; 0 0 0 1]  VectorParams1D=off
  Terminator : Terminator
  Tb3 : Outport
  PbLef : Outport  Port=2
  wires:
  Constant/1 -> Product1/2
  q[1...3]/1 -> T30/1(In1)
  T30/1(Out1) -> Product2/2
  Tbleg1/1 -> Product2/1
  Demux2/3 -> Mux/3
  Product1/1 -> Demux2/1
  Demux2/4 -> Terminator/1
  Demux2/1 -> Mux/1
  Mux/1 -> PbLef/1
  Demux2/2 -> Mux/2
  Product2/1 -> Tb3/1, Product1/1

== system hexapod/Forward Kinematic/TB3L6 ==
  note: Tb3
  note: PBL1ef
  q[1...3] : Inport
  Constant : Constant  Value=[L3; 0; 0; 1]  VectorParams1D=off
  Demux2 : Demux
  Mux : Mux  Inputs=3
  Product1 : Product  Multiplication=Matrix(*)
  Product2 : Product  Multiplication=Matrix(*)
  T30 : Subsystem
  Tbleg1 : Constant  Value=[cos(-135*pi/180) -sin(-135*pi/180) 0 -bL/2; sin(-135*pi/180) cos(-135*pi/180) 0 -bWs/2; 0 0 1 0; 0 0 0 1]  VectorParams1D=off
  Terminator : Terminator
  Tb3 : Outport
  PbLef : Outport  Port=2
  wires:
  Constant/1 -> Product1/2
  q[1...3]/1 -> T30/1(In1)
  T30/1(Out1) -> Product2/2
  Tbleg1/1 -> Product2/1
  Demux2/3 -> Mux/3
  Product1/1 -> Demux2/1
  Demux2/4 -> Terminator/1
  Demux2/1 -> Mux/1
  Mux/1 -> PbLef/1
  Demux2/2 -> Mux/2
  Product2/1 -> Tb3/1, Product1/1

== system hexapod/Forward Kinematic/TG31 ==
  note: PGL1ef
  TGb : Inport
  Tb3 : Inport  Port=2
  Constant1 : Constant  Value=[0; L3; 0; 1]  VectorParams1D=off
  Demux1 : Demux
  Mux1 : Mux  Inputs=3
  Product3 : Product  Multiplication=Matrix(*)
  Product4 : Product  Multiplication=Matrix(*)
  Terminator1 : Terminator
  PGLef : Outport
  wires:
  Tb3/1 -> Product3/2
  Demux1/2 -> Mux1/2
  Demux1/4 -> Terminator1/1
  Demux1/3 -> Mux1/3
  Mux1/1 -> PGLef/1
  Product4/1 -> Demux1/1
  Demux1/1 -> Mux1/1
  Constant1/1 -> Product4/2
  TGb/1 -> Product3/1
  Product3/1 -> Product4/1

== system hexapod/Forward Kinematic/TG32 ==
  note: PGL1ef
  TGb : Inport
  Tb3 : Inport  Port=2
  Constant1 : Constant  Value=[0; L3; 0; 1]  VectorParams1D=off
  Demux1 : Demux
  Mux1 : Mux  Inputs=3
  Product3 : Product  Multiplication=Matrix(*)
  Product4 : Product  Multiplication=Matrix(*)
  Terminator1 : Terminator
  PGLef : Outport
  wires:
  Product3/1 -> Product4/1
  TGb/1 -> Product3/1
  Constant1/1 -> Product4/2
  Demux1/1 -> Mux1/1
  Product4/1 -> Demux1/1
  Mux1/1 -> PGLef/1
  Demux1/3 -> Mux1/3
  Demux1/4 -> Terminator1/1
  Demux1/2 -> Mux1/2
  Tb3/1 -> Product3/2

== system hexapod/Forward Kinematic/TG33 ==
  note: PGL1ef
  TGb : Inport
  Tb3 : Inport  Port=2
  Constant1 : Constant  Value=[0; L3; 0; 1]  VectorParams1D=off
  Demux1 : Demux
  Mux1 : Mux  Inputs=3
  Product3 : Product  Multiplication=Matrix(*)
  Product4 : Product  Multiplication=Matrix(*)
  Terminator1 : Terminator
  PGLef : Outport
  wires:
  Tb3/1 -> Product3/2
  Demux1/2 -> Mux1/2
  Demux1/4 -> Terminator1/1
  Demux1/3 -> Mux1/3
  Mux1/1 -> PGLef/1
  Product4/1 -> Demux1/1
  Demux1/1 -> Mux1/1
  Constant1/1 -> Product4/2
  TGb/1 -> Product3/1
  Product3/1 -> Product4/1

== system hexapod/Forward Kinematic/TG34 ==
  note: PGL1ef
  TGb : Inport
  Tb3 : Inport  Port=2
  Constant1 : Constant  Value=[0; L3; 0; 1]  VectorParams1D=off
  Demux1 : Demux
  Mux1 : Mux  Inputs=3
  Product3 : Product  Multiplication=Matrix(*)
  Product4 : Product  Multiplication=Matrix(*)
  Terminator1 : Terminator
  PGLef : Outport
  wires:
  Product3/1 -> Product4/1
  TGb/1 -> Product3/1
  Constant1/1 -> Product4/2
  Demux1/1 -> Mux1/1
  Product4/1 -> Demux1/1
  Mux1/1 -> PGLef/1
  Demux1/3 -> Mux1/3
  Demux1/4 -> Terminator1/1
  Demux1/2 -> Mux1/2
  Tb3/1 -> Product3/2

== system hexapod/Forward Kinematic/TG35 ==
  note: PGL1ef
  TGb : Inport
  Tb3 : Inport  Port=2
  Constant1 : Constant  Value=[0; L3; 0; 1]  VectorParams1D=off
  Demux1 : Demux
  Mux1 : Mux  Inputs=3
  Product3 : Product  Multiplication=Matrix(*)
  Product4 : Product  Multiplication=Matrix(*)
  Terminator1 : Terminator
  PGLef : Outport
  wires:
  Tb3/1 -> Product3/2
  Demux1/2 -> Mux1/2
  Demux1/4 -> Terminator1/1
  Demux1/3 -> Mux1/3
  Mux1/1 -> PGLef/1
  Product4/1 -> Demux1/1
  Demux1/1 -> Mux1/1
  Constant1/1 -> Product4/2
  TGb/1 -> Product3/1
  Product3/1 -> Product4/1

== system hexapod/Forward Kinematic/TG36 ==
  note: PGL1ef
  TGb : Inport
  Tb3 : Inport  Port=2
  Constant1 : Constant  Value=[0; L3; 0; 1]  VectorParams1D=off
  Demux1 : Demux
  Mux1 : Mux  Inputs=3
  Product3 : Product  Multiplication=Matrix(*)
  Product4 : Product  Multiplication=Matrix(*)
  Terminator1 : Terminator
  PGLef : Outport
  wires:
  Tb3/1 -> Product3/2
  Demux1/2 -> Mux1/2
  Demux1/4 -> Terminator1/1
  Demux1/3 -> Mux1/3
  Mux1/1 -> PGLef/1
  Product4/1 -> Demux1/1
  Demux1/1 -> Mux1/1
  Constant1/1 -> Product4/2
  TGb/1 -> Product3/1
  Product3/1 -> Product4/1

== system hexapod/Gait Generator/Leg1_xyz ==
  Interpreted MATLAB Function : MATLABFcn  MATLABFcn=[u(1); u(2); u(3); 1]
  LEG1_X : simulink/Sources/Repeating Sequence Interpolated  OutValues=[l1x l1x-stX l1x-stX l1x+stX l1x+stX l1x].'  TimeValues=[0 0.25*Ts 0.375*Ts 0.625*Ts 0.75*Ts Ts].'  LookUpMeth=Interpolation-Use End Values  tsamp=0.01  OutMin=[]  OutMax=[]  OutDataTypeStr=double  OutputDataTypeScalingMode=double  OutDataType=fixdt(0,8)  OutScaling=2^-10
  LEG1_Y : Constant  Value=l1y
  LEG1_Z : simulink/Sources/Repeating Sequence Interpolated  OutValues="[l1z  l1z l1z+stZ l1z+stZ l1z l1z].'"  TimeValues=[0 0.25*Ts 0.375*Ts 0.625*Ts 0.75*Ts Ts].'  LookUpMeth=Interpolation-Use End Values  tsamp=0.01  OutMin=[]  OutMax=[]  OutDataTypeStr=double  OutputDataTypeScalingMode=double  OutDataType=fixdt(0,8)  OutScaling=2^-10
  Mux : Mux  Inputs=3
  Scope6 : Scope  NumInputPorts=3
      settings: YMin=-15~-5~-5  YMax=20~5~5  SaveName=ScopeData15
  Out1 : Outport
  wires:
  LEG1_Z/1 -> Scope6/3, Mux/3
  LEG1_Y/1 -> Scope6/2, Mux/2
  LEG1_X/1 -> Scope6/1, Mux/1
  Mux/1 -> Interpreted MATLAB Function/1
  Interpreted MATLAB Function/1 -> Out1/1

== system hexapod/Gait Generator/Leg2_xyz ==
  Interpreted MATLAB Function1 : MATLABFcn  MATLABFcn=[u(1); u(2); u(3); 1]
  LEG2_X : simulink/Sources/Repeating Sequence Interpolated  OutValues=[l2x l2x+stX l2x+stX l2x-stX l2x-stX l2x].'  TimeValues=[0 0.125*Ts 0.25*Ts 0.75*Ts 0.875*Ts Ts].'  LookUpMeth=Interpolation-Use End Values  tsamp=0.01  OutMin=[]  OutMax=[]  OutDataTypeStr=double  OutputDataTypeScalingMode=double  OutDataType=fixdt(0,8)  OutScaling=2^-10
  LEG2_Y : Constant  Value=l2y
  LEG2_Z : simulink/Sources/Repeating Sequence Interpolated  OutValues=[l2z+stZ l2z+stZ l2z l2z l2z+stZ l2z+stZ].'  TimeValues=[0 0.125*Ts 0.25*Ts 0.75*Ts 0.875*Ts Ts].'  LookUpMeth=Interpolation-Use End Values  tsamp=0.01  OutMin=[]  OutMax=[]  OutDataTypeStr=double  OutputDataTypeScalingMode=double  OutDataType=fixdt(0,8)  OutScaling=2^-10
  Mux1 : Mux  Inputs=3
  Scope6 : Scope  NumInputPorts=3
      settings: YMin=-15~-5~-5  YMax=20~5~5  SaveName=ScopeData40
  Out1 : Outport
  wires:
  LEG2_Z/1 -> Scope6/3, Mux1/3
  LEG2_X/1 -> Scope6/1, Mux1/1
  Mux1/1 -> Interpreted MATLAB Function1/1
  Interpreted MATLAB Function1/1 -> Out1/1
  LEG2_Y/1 -> Scope6/2, Mux1/2

== system hexapod/Gait Generator/Leg3_xyz ==
  Interpreted MATLAB Function2 : MATLABFcn  MATLABFcn=[u(1); u(2); u(3); 1]
  LEG3_X : simulink/Sources/Repeating Sequence Interpolated  OutValues=[l3x l3x-stX l3x-stX l3x+stX l3x+stX l3x].'  TimeValues=[0 0.25*Ts 0.375*Ts 0.625*Ts 0.75*Ts Ts].'  LookUpMeth=Interpolation-Use End Values  tsamp=0.01  OutMin=[]  OutMax=[]  OutDataTypeStr=double  OutputDataTypeScalingMode=double  OutDataType=fixdt(0,8)  OutScaling=2^-10
  LEG3_Y : Constant  Value=l3y
  LEG3_Z : simulink/Sources/Repeating Sequence Interpolated  OutValues="[l3z  l3z l3z+stZ l3z+stZ l3z l3z].'"  TimeValues=[0 0.25*Ts 0.375*Ts 0.625*Ts 0.75*Ts Ts].'  LookUpMeth=Interpolation-Use End Values  tsamp=0.01  OutMin=[]  OutMax=[]  OutDataTypeStr=double  OutputDataTypeScalingMode=double  OutDataType=fixdt(0,8)  OutScaling=2^-10
  Mux2 : Mux  Inputs=3
  Scope6 : Scope  NumInputPorts=3
      settings: YMin=-15~-5~-5  YMax=20~5~5  SaveName=ScopeData41
  Out1 : Outport
  wires:
  Mux2/1 -> Interpreted MATLAB Function2/1
  Interpreted MATLAB Function2/1 -> Out1/1
  LEG3_X/1 -> Scope6/1, Mux2/1
  LEG3_Z/1 -> Scope6/3, Mux2/3
  LEG3_Y/1 -> Scope6/2, Mux2/2

== system hexapod/Gait Generator/Leg4_xyz ==
  Interpreted MATLAB Function3 : MATLABFcn  MATLABFcn=[u(1); u(2); u(3); 1]
  LEG4_X : simulink/Sources/Repeating Sequence Interpolated  OutValues=[l4x l4x+stX l4x+stX l4x-stX l4x-stX l4x].'  TimeValues=[0 0.125*Ts 0.25*Ts 0.75*Ts 0.875*Ts Ts].'  LookUpMeth=Interpolation-Use End Values  tsamp=0.01  OutMin=[]  OutMax=[]  OutDataTypeStr=double  OutputDataTypeScalingMode=double  OutDataType=fixdt(0,8)  OutScaling=2^-10
  LEG4_Y : Constant  Value=l4y
  LEG4_Z : simulink/Sources/Repeating Sequence Interpolated  OutValues=[l4z+stZ l4z+stZ l4z l4z l4z+stZ l4z+stZ].'  TimeValues=[0 0.125*Ts 0.25*Ts 0.75*Ts 0.875*Ts Ts].'  LookUpMeth=Interpolation-Use End Values  tsamp=0.01  OutMin=[]  OutMax=[]  OutDataTypeStr=double  OutputDataTypeScalingMode=double  OutDataType=fixdt(0,8)  OutScaling=2^-10
  Mux3 : Mux  Inputs=3
  Scope6 : Scope  NumInputPorts=3
      settings: YMin=-15~-5~-5  YMax=20~5~5  SaveName=ScopeData42
  Out1 : Outport
  wires:
  Mux3/1 -> Interpreted MATLAB Function3/1
  LEG4_X/1 -> Scope6/1, Mux3/1
  Interpreted MATLAB Function3/1 -> Out1/1
  LEG4_Y/1 -> Scope6/2, Mux3/2
  LEG4_Z/1 -> Scope6/3, Mux3/3

== system hexapod/Gait Generator/Leg5_xyz ==
  Interpreted MATLAB Function4 : MATLABFcn  MATLABFcn=[u(1); u(2); u(3); 1]
  LEG5_X : simulink/Sources/Repeating Sequence Interpolated  OutValues=[l5x l5x-stX l5x-stX l5x+stX l5x+stX l5x].'  TimeValues=[0 0.25*Ts 0.375*Ts 0.625*Ts 0.75*Ts Ts].'  LookUpMeth=Interpolation-Use End Values  tsamp=0.01  OutMin=[]  OutMax=[]  OutDataTypeStr=double  OutputDataTypeScalingMode=double  OutDataType=fixdt(0,8)  OutScaling=2^-10
  LEG5_Y : Constant  Value=l5y
  LEG5_Z : simulink/Sources/Repeating Sequence Interpolated  OutValues="[l5z  l5z l5z+stZ l5z+stZ l5z l5z].'"  TimeValues=[0 0.25*Ts 0.375*Ts 0.625*Ts 0.75*Ts Ts].'  LookUpMeth=Interpolation-Use End Values  tsamp=0.01  OutMin=[]  OutMax=[]  OutDataTypeStr=double  OutputDataTypeScalingMode=double  OutDataType=fixdt(0,8)  OutScaling=2^-10
  Mux4 : Mux  Inputs=3
  Scope6 : Scope  NumInputPorts=3
      settings: YMin=-15~-5~-5  YMax=20~5~5  SaveName=ScopeData8
  Out1 : Outport
  wires:
  LEG5_X/1 -> Scope6/1, Mux4/1
  LEG5_Y/1 -> Scope6/2, Mux4/2
  Interpreted MATLAB Function4/1 -> Out1/1
  LEG5_Z/1 -> Scope6/3, Mux4/3
  Mux4/1 -> Interpreted MATLAB Function4/1

== system hexapod/Gait Generator/Leg6_xyz ==
  Interpreted MATLAB Function5 : MATLABFcn  MATLABFcn=[u(1); u(2); u(3); 1]
  LEG6_X : simulink/Sources/Repeating Sequence Interpolated  OutValues=[l6x l6x+stX l6x+stX l6x-stX l6x-stX l6x].'  TimeValues=[0 0.125*Ts 0.25*Ts 0.75*Ts 0.875*Ts Ts].'  LookUpMeth=Interpolation-Use End Values  tsamp=0.01  OutMin=[]  OutMax=[]  OutDataTypeStr=double  OutputDataTypeScalingMode=double  OutDataType=fixdt(0,8)  OutScaling=2^-10
  LEG6_Y : Constant  Value=l6y
  LEG6_Z : simulink/Sources/Repeating Sequence Interpolated  OutValues=[l6z+stZ l6z+stZ l6z l6z l6z+stZ l6z+stZ].'  TimeValues=[0 0.125*Ts 0.25*Ts 0.75*Ts 0.875*Ts Ts].'  LookUpMeth=Interpolation-Use End Values  tsamp=0.01  OutMin=[]  OutMax=[]  OutDataTypeStr=double  OutputDataTypeScalingMode=double  OutDataType=fixdt(0,8)  OutScaling=2^-10
  Mux5 : Mux  Inputs=3
  Scope6 : Scope  NumInputPorts=3
      settings: YMin=-15~-5~-5  YMax=20~5~5  SaveName=ScopeData10
  Out1 : Outport
  wires:
  LEG6_Y/1 -> Scope6/2, Mux5/2
  LEG6_Z/1 -> Scope6/3, Mux5/3
  LEG6_X/1 -> Scope6/1, Mux5/1
  Interpreted MATLAB Function5/1 -> Out1/1
  Mux5/1 -> Interpreted MATLAB Function5/1

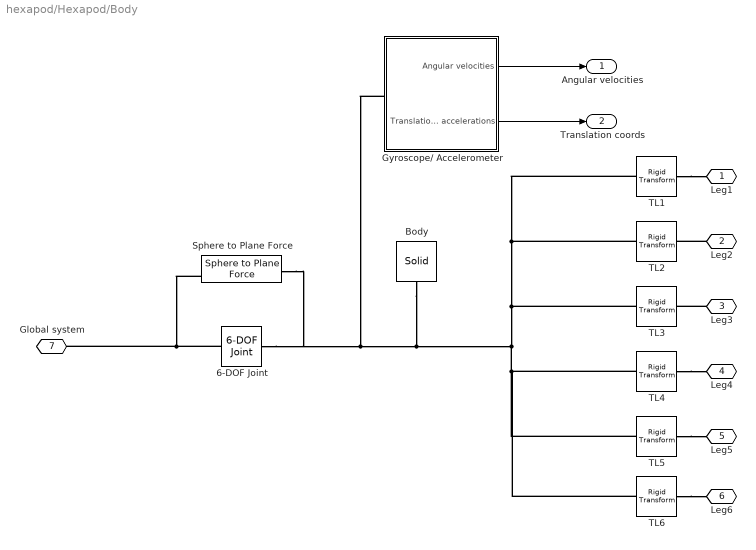
== system hexapod/Hexapod/Body ==
  6-DOF Joint : sm_lib/Joints/6-DOF Joint  SenseConstraintForce=off  SenseConstraintForceX=off  SenseConstraintForceY=off  SenseConstraintForceZ=off  SenseConstraintTorque=off  SenseConstraintTorqueX=off  SenseConstraintTorqueY=off  SenseConstraintTorqueZ=off  SenseTotalForce=off  SenseTotalForceX=off  SenseTotalForceY=off  SenseTotalForceZ=off  SenseTotalTorque=off  SenseTotalTorqueX=off  SenseTotalTorqueY=off  SenseTotalTorqueZ=off  CompositeWrenchDir=FollowerOnBase  CompositeWrenchFrame=BaseFrame  PxEquilibriumPosition=0  PxEquilibriumPositionUnits=m  PxSpringStiffness=0  PxSpringStiffnessUnits=N/m  PxDampingCoefficient=0  PxDampingCoefficientUnits=N/(m/s)  PxTorqueActuationMode=NoTorque  PxMotionActuationMode=ComputedMotion  PxSensePosition=off  PxSenseVelocity=off  PxSenseAcceleration=off  PxSenseTorqueForce=off  PxPositionTargetSpecify=off  PxPositionTargetPriority=High  PxPositionTargetValue=0.5  PxPositionTargetValueUnits=m  PxVelocityTargetSpecify=off  PxVelocityTargetPriority=High  PxVelocityTargetValue=0.5  PxVelocityTargetValueUnits=m/s  PyEquilibriumPosition=0  PyEquilibriumPositionUnits=m  PySpringStiffness=0  PySpringStiffnessUnits=N/m  PyDampingCoefficient=0  PyDampingCoefficientUnits=N/(m/s)  PyTorqueActuationMode=NoTorque  PyMotionActuationMode=ComputedMotion  PySensePosition=off  PySenseVelocity=off  PySenseAcceleration=off  PySenseTorqueForce=off  PyPositionTargetSpecify=off  PyPositionTargetPriority=High  PyPositionTargetValue=0  PyPositionTargetValueUnits=m  PyVelocityTargetSpecify=off  PyVelocityTargetPriority=High  PyVelocityTargetValue=0  PyVelocityTargetValueUnits=m/s  PzEquilibriumPosition=0  PzEquilibriumPositionUnits=m  PzSpringStiffness=0  PzSpringStiffnessUnits=N/m  PzDampingCoefficient=0  PzDampingCoefficientUnits=N/(m/s)  PzTorqueActuationMode=NoTorque  PzMotionActuationMode=ComputedMotion  PzSensePosition=off  PzSenseVelocity=off  PzSenseAcceleration=off  PzSenseTorqueForce=off  PzPositionTargetSpecify=on  PzPositionTargetPriority=High  PzPositionTargetValue=0.2  PzPositionTargetValueUnits=m  PzVelocityTargetSpecify=off  PzVelocityTargetPriority=High  PzVelocityTargetValue=0  PzVelocityTargetValueUnits=m/s  SphDefPosRotationMethod=None  SphDefPosRotationAngleUnits=deg  SphDefPosRotationStandardAxis=+Z  SphDefPosRotationAngle=0.0  SphDefPosRotationArbitraryAxis=[0 0 1]  SphDefPosFollAlignAxisA=+X  SphDefPosBaseAlignAxisA=+Y  SphDefPosFollAlignAxisB=+Y  SphDefPosBaseAlignAxisB=+Z  SphDefPosRotationMatrix=[1 0 0; 0 1 0; 0 0 1]  SphEqPosRotationMethod=None  SphEqPosRotationAngleUnits=deg  SphEqPosRotationStandardAxis=+Z  SphEqPosRotationAngle=0.0  SphEqPosRotationArbitraryAxis=[0 0 1]  SphEqPosFollAlignAxisA=+X  SphEqPosBaseAlignAxisA=+Y  SphEqPosFollAlignAxisB=+Y  SphEqPosBaseAlignAxisB=+Z  SphEqPosRotationMatrix=[1 0 0; 0 1 0; 0 0 1]  SphSpringStiffness=0  SphSpringStiffnessUnits=N*m/deg  SphDampingCoefficient=0  SphDampingCoefficientUnits=N*m/(deg/s)  SphActuateTorqueX=off  SphActuateTorqueY=off  SphActuateTorqueZ=off  SphActuateTorque=off  SphTorqueActuationMode=NoTorque  SphMotionActuationMode=ComputedMotion  SphActuationFrame=BaseFrame  SphSensePosition=off  SphSenseVelocityX=off  SphSenseVelocityY=off  SphSenseVelocityZ=off  SphSenseVelocity=off  SphSenseAccelerationX=off  SphSenseAccelerationY=off  SphSenseAccelerationZ=off  SphSenseAcceleration=off  SphSenseTorqueX=off  SphSenseTorqueY=off  SphSenseTorqueZ=off  SphSenseTorqueForce=off  SphSensingFrame=BaseFrame  SphPositionTargetRotationMethod=None  SphPositionTargetRotationAngleUnits=deg  SphPositionTargetRotationStandardAxis=+Z  SphPositionTargetRotationAngle=0.0  SphPositionTargetRotationArbitraryAxis=[0 0 1]  SphPositionTargetFollAlignAxisA=+X  SphPositionTargetBaseAlignAxisA=+Y  SphPositionTargetFollAlignAxisB=+Y  SphPositionTargetBaseAlignAxisB=+Z  SphPositionTargetRotationMatrix=[1 0 0; 0 1 0; 0 0 1]  SphPositionTargetSpecify=off  SphPositionTargetPriority=High  SphVelocityTargetValue=[0 0 0]  SphVelocityTargetValueUnits=deg/s  SphVelocityTargetSpecify=off  SphVelocityTargetPriority=High  SphVelocityTargetInFollowerFrame=on  BlockFunction=simmechanics.library.joints.sixdof_joint
  Body : sm_lib/Body Elements/Solid  InertiaType=CalculateFromGeometry  Mass=m  MassUnits=kg  CenterOfMass=[0 0 0]  CenterOfMassUnits=m  MomentsOfInertia=[1 1 1]  MomentsOfInertiaUnits=kg*m^2  ProductsOfInertia=[0 0 0]  ProductsOfInertiaUnits=kg*m^2  DensityBased=off  Density=5000  DensityUnits=kg/(m^3)  GraphicType=FromGeometry  MarkerShape=Sphere  MarkerSize=10  MarkerSizeUnits=m  GraphicVisPropType=SimpleVisualProperties  GraphicDiffuseColor=[0.0 0.4 0.0]  GraphicSpecularColor=[0.5 0.5 0.5 1.0]  GraphicAmbientColor=[0.15 0.15 0.15 1.0]  GraphicEmissiveColor=[0.0 0.0 0.0 1.0]  GraphicShininess=75  GraphicOpacity=1.0  GeometryShape=FromFile  RectangleSize=[1 1]  RectangleSizeUnits=m  BrickDimensions=[18.5 12.5 1]  BrickDimensionUnits=cm  CylinderRadius=1  CylinderRadiusUnits=m  CylinderLength=1  CylinderLengthUnits=m  SphereRadius=1  SphereRadiusUnits=m  EllipsoidRadii=[1 1 1]  EllipsoidRadiiUnits=m  ExtrusionCrossSection=[L/2 w1/2; 0 w2/2; -L/2 w1/2; -L/2 -w1/2; 0 -w2/2; L/2 -w1/2]  ExtrusionCrossSectionUnits=cm  ExtrusionLength=H  ExtrusionLengthUnits=cm  PolygonNumSides=3  PolygonOuterRadius=1  PolygonOuterRadiusUnits=m  ExtGeomFileType=STEP  ExtGeomFileName=D:\Институт\Высертация\Model\3d\Body.STEP  ExtGeomFileUnits=m  RevolutionCrossSection=[1 1; 1 -1; 2 -1; 2 1]  RevolutionCrossSectionUnits=m  RevolutionExtent=Full  RevolutionAngle=180  RevolutionAngleUnits=deg  BlockFunction=simmechanics.library.body_elements.solid
  Gyroscope/ Accelerometer : Subsystem
  Sphere to Plane Force : Contact_Forces_Lib/3D/Sphere to Plane Force  sphere_rad=0.005  plane_lenx=GsurfX  plane_leny=GsurfY  plane_depth=0.01/2  force_law=Linear  k_contact=1e7  b_contact=1e4  pen_full_damp_F=1e-4  pen_exponent=1  custom_param_1=1  custom_param_2=1  friction_law=None  mu_kinetic=0.5  mu_static=0.7  v_thr=0.001
  TL1 : sm_lib/Frames and Transforms/Rigid Transform  TranslationMethod=Cartesian  TranslationLengthUnit=cm  TranslationStandardAxis=+Z  TranslationStandardOffset=0  TranslationCartesianOffset=[L/2 w1/2 0]  TranslationROffset=0  TranslationROffsetUnits=m  TranslationZOffset=0  TranslationZOffsetUnits=m  TranslationThetaOffset=0  TranslationThetaOffsetUnits=deg  RotationMethod=StandardAxis  RotationAngleUnits=deg  RotationStandardAxis=+Z  RotationAngle=90-Z1Angle  RotationArbitraryAxis=[0 0 1]  FollAlignAxisA=+X  BaseAlignAxisA=+Y  FollAlignAxisB=+Y  BaseAlignAxisB=+Z  RotationMatrix=[1 0 0; 0 1 0; 0 0 1]  BlockFunction=simmechanics.library.frames_transforms.rigid_transform
  TL2 : sm_lib/Frames and Transforms/Rigid Transform  TranslationMethod=Cartesian  TranslationLengthUnit=cm  TranslationStandardAxis=+Z  TranslationStandardOffset=0  TranslationCartesianOffset=[0 w2/2 0]  TranslationROffset=0  TranslationROffsetUnits=m  TranslationZOffset=0  TranslationZOffsetUnits=m  TranslationThetaOffset=0  TranslationThetaOffsetUnits=deg  RotationMethod=StandardAxis  RotationAngleUnits=deg  RotationStandardAxis=+Z  RotationAngle=90-Z2Angle  RotationArbitraryAxis=[0 0 1]  FollAlignAxisA=+X  BaseAlignAxisA=+Y  FollAlignAxisB=+Y  BaseAlignAxisB=+Z  RotationMatrix=[1 0 0; 0 1 0; 0 0 1]  BlockFunction=simmechanics.library.frames_transforms.rigid_transform
  TL3 : sm_lib/Frames and Transforms/Rigid Transform  TranslationMethod=Cartesian  TranslationLengthUnit=cm  TranslationStandardAxis=+Z  TranslationStandardOffset=0  TranslationCartesianOffset=[-L/2 w1/2 0]  TranslationROffset=0  TranslationROffsetUnits=m  TranslationZOffset=0  TranslationZOffsetUnits=m  TranslationThetaOffset=0  TranslationThetaOffsetUnits=deg  RotationMethod=StandardAxis  RotationAngleUnits=deg  RotationStandardAxis=+Z  RotationAngle=90-Z3Angle  RotationArbitraryAxis=[0 0 1]  FollAlignAxisA=+X  BaseAlignAxisA=+Y  FollAlignAxisB=+Y  BaseAlignAxisB=+Z  RotationMatrix=[1 0 0; 0 1 0; 0 0 1]  BlockFunction=simmechanics.library.frames_transforms.rigid_transform
  TL4 : sm_lib/Frames and Transforms/Rigid Transform  TranslationMethod=Cartesian  TranslationLengthUnit=cm  TranslationStandardAxis=+Z  TranslationStandardOffset=0  TranslationCartesianOffset=[L/2 -w1/2 0]  TranslationROffset=0  TranslationROffsetUnits=m  TranslationZOffset=0  TranslationZOffsetUnits=m  TranslationThetaOffset=0  TranslationThetaOffsetUnits=deg  RotationMethod=StandardAxis  RotationAngleUnits=deg  RotationStandardAxis=+Z  RotationAngle=-90-Z4Angle  RotationArbitraryAxis=[0 0 1]  FollAlignAxisA=+X  BaseAlignAxisA=+Y  FollAlignAxisB=+Y  BaseAlignAxisB=+Z  RotationMatrix=[1 0 0; 0 1 0; 0 0 1]  BlockFunction=simmechanics.library.frames_transforms.rigid_transform
  TL5 : sm_lib/Frames and Transforms/Rigid Transform  TranslationMethod=Cartesian  TranslationLengthUnit=cm  TranslationStandardAxis=+Z  TranslationStandardOffset=0  TranslationCartesianOffset=[0 -w2/2 0]  TranslationROffset=0  TranslationROffsetUnits=m  TranslationZOffset=0  TranslationZOffsetUnits=m  TranslationThetaOffset=0  TranslationThetaOffsetUnits=deg  RotationMethod=StandardAxis  RotationAngleUnits=deg  RotationStandardAxis=+Z  RotationAngle=-90-Z5Angle  RotationArbitraryAxis=[0 0 1]  FollAlignAxisA=+X  BaseAlignAxisA=+Y  FollAlignAxisB=+Y  BaseAlignAxisB=+Z  RotationMatrix=[1 0 0; 0 1 0; 0 0 1]  BlockFunction=simmechanics.library.frames_transforms.rigid_transform
  TL6 : sm_lib/Frames and Transforms/Rigid Transform  TranslationMethod=Cartesian  TranslationLengthUnit=cm  TranslationStandardAxis=+Z  TranslationStandardOffset=0  TranslationCartesianOffset=[-L/2 -w1/2 0]  TranslationROffset=0  TranslationROffsetUnits=m  TranslationZOffset=0  TranslationZOffsetUnits=m  TranslationThetaOffset=0  TranslationThetaOffsetUnits=deg  RotationMethod=StandardAxis  RotationAngleUnits=deg  RotationStandardAxis=+Z  RotationAngle=-90-Z6Angle  RotationArbitraryAxis=[0 0 1]  FollAlignAxisA=+X  BaseAlignAxisA=+Y  FollAlignAxisB=+Y  BaseAlignAxisB=+Z  RotationMatrix=[1 0 0; 0 1 0; 0 0 1]  BlockFunction=simmechanics.library.frames_transforms.rigid_transform
  Leg1 : PMIOPort  Port=1  Side=Left
  Leg2 : PMIOPort  Port=2  Side=Left
  Leg3 : PMIOPort  Port=3  Side=Left
  Leg4 : PMIOPort  Port=4  Side=Right
  Leg5 : PMIOPort  Port=5  Side=Right
  Leg6 : PMIOPort  Port=6  Side=Right
  Global system : PMIOPort  Port=7  Side=Left
  Angular velocities : Outport
  Translation coords : Outport  Port=2
  wires:
  Gyroscope/ Accelerometer/1(Angular velocities) -> Angular velocities/1
  Gyroscope/ Accelerometer/2(Translation accelerations) -> Translation coords/1
  connections:
  TL1/RConn1 -- Leg1/RConn1
  Leg2/RConn1 -- TL2/RConn1
  Leg3/RConn1 -- TL3/RConn1
  TL4/RConn1 -- Leg4/RConn1
  TL5/RConn1 -- Leg5/RConn1
  TL6/RConn1 -- Leg6/RConn1
  TL1/LConn1 -- Gyroscope/ Accelerometer/LConn1 -- Sphere to Plane Force/LConn1 -- 6-DOF Joint/RConn1 -- Body/RConn1 -- TL6/LConn1 -- TL5/LConn1 -- TL4/LConn1 -- TL3/LConn1 -- TL2/LConn1
  6-DOF Joint/LConn1 -- Sphere to Plane Force/RConn1 -- Global system/RConn1
